simulink model "block190118_1"  (R2018a)
settings: Solver=ode4  StartTime=0.0  StopTime=10  FixedStep=0.1  RelTol=1e-3
libraries: dspsrcs4 x1
settings Model: Creator=Kenneth  LastModifiedBy=Kenneth
settings SolverCC: AutoInsertRateTranBlk=on
settings DataIOCC: LimitDataPoints=on  SaveOutput=off  SignalLogging=off  SaveTime=off
settings OptimizationCC: LifeSpan=inf
settings DebuggingCC: AlgebraicLoopMsg=error  SingleTaskRateTransMsg=error  AllowSymbolicDim=off  SFUnexpectedBacktrackingDiag=warning  SFNoUnconditionalDefaultTransitionDiag=warning  SFExecutionAtInitializationDiag=none
settings CodeAppCC: StateflowObjectComments=on
settings GRTTargetCC: TargetLangStandard=C89/C90 (ANSI)  GeneratePreprocessorConditionals=Disable all

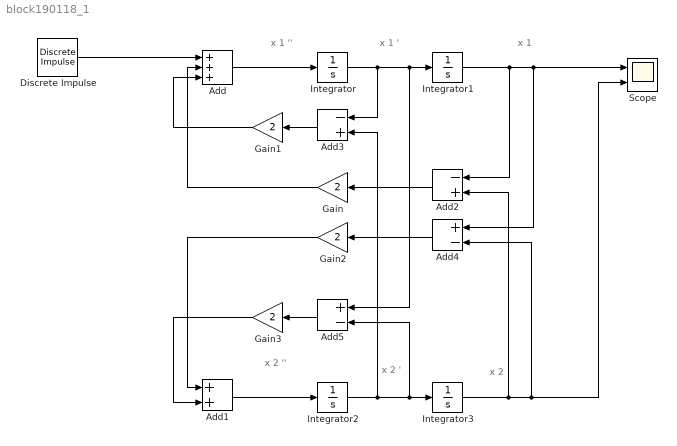
== system block190118_1 ==
  note: x 2
  note: x 2 '
  note: x 2 ''
  note: x 1
  note: x 1 '
  note: x 1 ''
  Add : Sum  Inputs=+++
  Add1 : Sum
  Add2 : Sum  Inputs=-+
  Add3 : Sum  Inputs=-+
  Add4 : Sum  Inputs=+-
  Add5 : Sum  Inputs=+-
  Discrete Impulse : dspsrcs4/Discrete  Impulse  Delay=1  SampleTime=1  FrameSample=1  OutputFrames=off  dataType=double  isSigned=on  wordLen=16  udDataType=sfix(16)  fracBitsMode=Best precision  numFracBits=15  OutDataTypeStr=double  LastOutDataTypeStr=double
  Gain{,1..3} (4 alike) : Gain  Gain=2
  Integrator{,1..3} (4 alike) : Integrator
  Scope : Scope  NumInputPorts=2
  wires:
  Add/1 -> Integrator/1
  Integrator1/1 -> Add2/1, Add4/1, Scope/1
  Add1/1 -> Integrator2/1
  Integrator2/1 -> Add3/2, Add5/2, Integrator3/1
  Integrator3/1 -> Add2/2, Add4/2, Scope/2
  Add2/1 -> Gain/1
  Gain/1 -> Add/2
  Integrator/1 -> Add3/1, Add5/1, Integrator1/1
  Add3/1 -> Gain1/1
  Gain1/1 -> Add/3
  Add4/1 -> Gain2/1
  Gain2/1 -> Add1/1
  Add5/1 -> Gain3/1
  Gain3/1 -> Add1/2
  Discrete Impulse/1 -> Add/1
